simulink model "TST_TIntkVUs_VD"  (R2016b)
settings: Solver=FixedStepDiscrete  StartTime=0.0  StopTime=simTime  FixedStep=sampleTime  RelTol=1e-3
values from neighbouring files (symbols this model uses):
  testCase = 1    [initTST_TIntkVUs_VD_001.m]    (also in initTST_TIntkVUs_VD_002.m = 2; initTST_TIntkVUs_VD_003.m = 3)
libraries: UnitTest_Lib x6, simulink x4
settings Model: Creator=liangyunbo  LastModifiedBy=liangyunbo
settings DebuggingCC: SignalRangeChecking=error

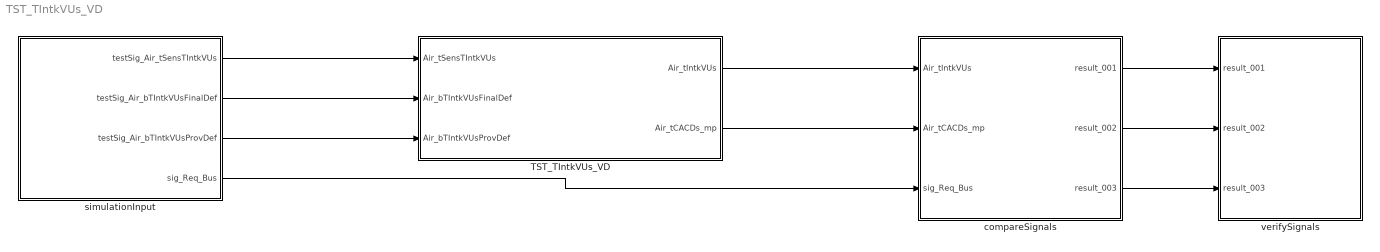
== system TST_TIntkVUs_VD ==
  TST_TIntkVUs_VD : Subsystem
  compareSignals : Subsystem
  simulationInput : Subsystem
  verifySignals : Subsystem
  wires:
  simulationInput/1(testSig_Air_tSensTIntkVUs) -> TST_TIntkVUs_VD/1(Air_tSensTIntkVUs)
  simulationInput/2(testSig_Air_bTIntkVUsFinalDef) -> TST_TIntkVUs_VD/2(Air_bTIntkVUsFinalDef)
  simulationInput/3(testSig_Air_bTIntkVUsProvDef) -> TST_TIntkVUs_VD/3(Air_bTIntkVUsProvDef)
  TST_TIntkVUs_VD/1(Air_tIntkVUs) -> compareSignals/1(Air_tIntkVUs)
  TST_TIntkVUs_VD/2(Air_tCACDs_mp) -> compareSignals/2(Air_tCACDs_mp)
  simulationInput/4(sig_Req_Bus) -> compareSignals/3(sig_Req_Bus)
  compareSignals/1(result_001) -> verifySignals/1(result_001)
  compareSignals/2(result_002) -> verifySignals/2(result_002)
  compareSignals/3(result_003) -> verifySignals/3(result_003)

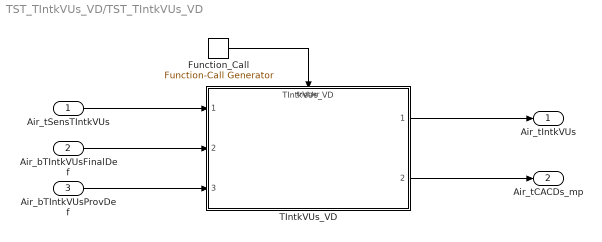
== system TST_TIntkVUs_VD/TST_TIntkVUs_VD ==
  Air_tSensTIntkVUs : Inport
  Air_bTIntkVUsFinalDef : Inport  Port=2
  Air_bTIntkVUsProvDef : Inport  Port=3
  Function_Call : simulink/Ports & Subsystems/Function-Call Generator  sample_time=sampleTime  numberOfIterations=1
  TIntkVUs_VD : ModelReference  ModelNameDialog=TIntkVUs_VD  SimulationMode=Normal  ModelReferenceVersion=1.16  TriggerPortName=function  TriggerPortTriggerType=function-call  TriggerPortStatesWhenEnabling=held
  Air_tIntkVUs : Outport
  Air_tCACDs_mp : Outport  Port=2
  wires:
  Function_Call/1 -> TIntkVUs_VD/Trigger
  Air_tSensTIntkVUs/1 -> TIntkVUs_VD/1
  Air_bTIntkVUsFinalDef/1 -> TIntkVUs_VD/2
  Air_bTIntkVUsProvDef/1 -> TIntkVUs_VD/3
  TIntkVUs_VD/1 -> Air_tIntkVUs/1
  TIntkVUs_VD/2 -> Air_tCACDs_mp/1

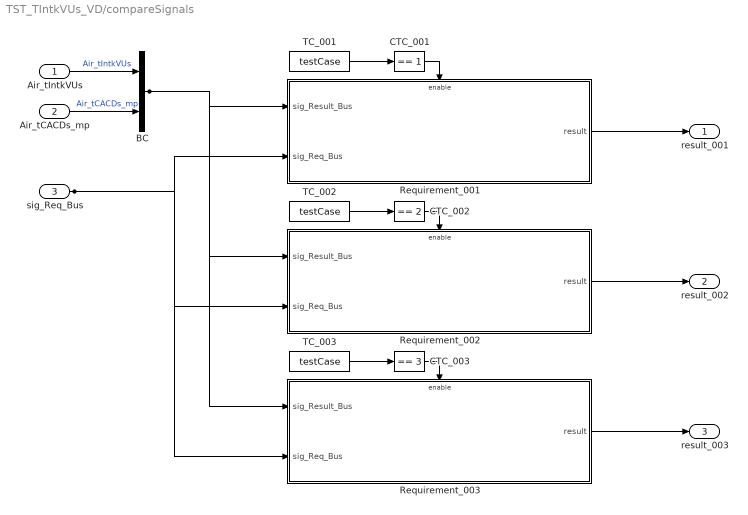
== system TST_TIntkVUs_VD/compareSignals ==
  Air_tIntkVUs : Inport
  Air_tCACDs_mp : Inport  Port=2
  sig_Req_Bus : Inport  Port=3
  BC : BusCreator  Inputs=2
  CTC_001 : simulink/Logic and Bit Operations/Compare To Constant  relop===  const=1  OutDataTypeStr=boolean
  CTC_002 : simulink/Logic and Bit Operations/Compare To Constant  relop===  const=2  OutDataTypeStr=boolean
  CTC_003 : simulink/Logic and Bit Operations/Compare To Constant  relop===  const=3  OutDataTypeStr=boolean
  Requirement_001 : Subsystem
  Requirement_002 : Subsystem
  Requirement_003 : Subsystem
  TC_001 : Constant  Value=testCase
  TC_002 : Constant  Value=testCase
  TC_003 : Constant  Value=testCase
  result_001 : Outport
  result_002 : Outport  Port=2
  result_003 : Outport  Port=3
  wires:
  Air_tIntkVUs/1 -> BC/1  "Air_tIntkVUs"
  Air_tCACDs_mp/1 -> BC/2  "Air_tCACDs_mp"
  TC_001/1 -> CTC_001/1
  CTC_001/1 -> Requirement_001/Enable
  sig_Req_Bus/1 -> Requirement_001/2(sig_Req_Bus), Requirement_002/2(sig_Req_Bus), Requirement_003/2(sig_Req_Bus)
  BC/1 -> Requirement_001/1(sig_Result_Bus), Requirement_002/1(sig_Result_Bus), Requirement_003/1(sig_Result_Bus)
  Requirement_001/1(result) -> result_001/1
  TC_002/1 -> CTC_002/1
  CTC_002/1 -> Requirement_002/Enable
  Requirement_002/1(result) -> result_002/1
  TC_003/1 -> CTC_003/1
  CTC_003/1 -> Requirement_003/Enable
  Requirement_003/1(result) -> result_003/1

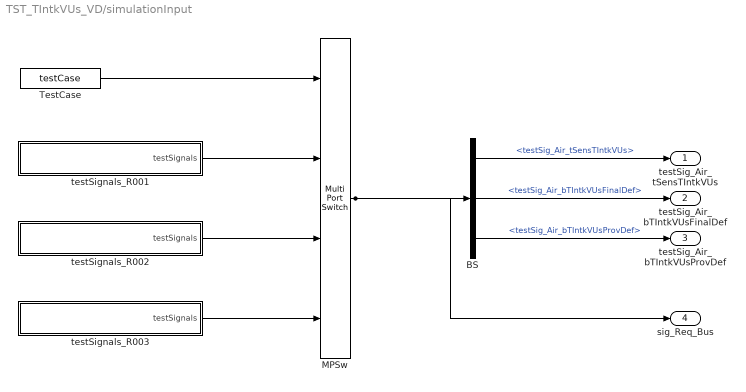
== system TST_TIntkVUs_VD/simulationInput ==
  BS : BusSelector  OutputSignals=testSig_Air_tSensTIntkVUs,testSig_Air_bTIntkVUsFinalDef,testSig_Air_bTIntkVUsProvDef
  MPSw : MultiPortSwitch  SaturateOnIntegerOverflow=on  InputSameDT=on
  TestCase : Constant  Value=testCase
  testSignals_R001 : Subsystem
  testSignals_R002 : Subsystem
  testSignals_R003 : Subsystem
  testSig_Air_tSensTIntkVUs : Outport
  testSig_Air_bTIntkVUsFinalDef : Outport  Port=2
  testSig_Air_bTIntkVUsProvDef : Outport  Port=3
  sig_Req_Bus : Outport  Port=4
  wires:
  BS/1 -> testSig_Air_tSensTIntkVUs/1  "<testSig_Air_tSensTIntkVUs>"
  BS/2 -> testSig_Air_bTIntkVUsFinalDef/1  "<testSig_Air_bTIntkVUsFinalDef>"
  BS/3 -> testSig_Air_bTIntkVUsProvDef/1  "<testSig_Air_bTIntkVUsProvDef>"
  MPSw/1 -> BS/1, sig_Req_Bus/1
  TestCase/1 -> MPSw/1
  testSignals_R001/1(testSignals) -> MPSw/2
  testSignals_R002/1(testSignals) -> MPSw/3
  testSignals_R003/1(testSignals) -> MPSw/4

== system TST_TIntkVUs_VD/verifySignals ==
  result_001 : Inport
  result_002 : Inport  Port=2
  result_003 : Inport  Port=3
  Assertion_001 : Assertion  Enabled=off
  Assertion_002 : Assertion  Enabled=off
  Assertion_003 : Assertion  Enabled=off
  wires:
  result_001/1 -> Assertion_001/1
  result_002/1 -> Assertion_002/1
  result_003/1 -> Assertion_003/1

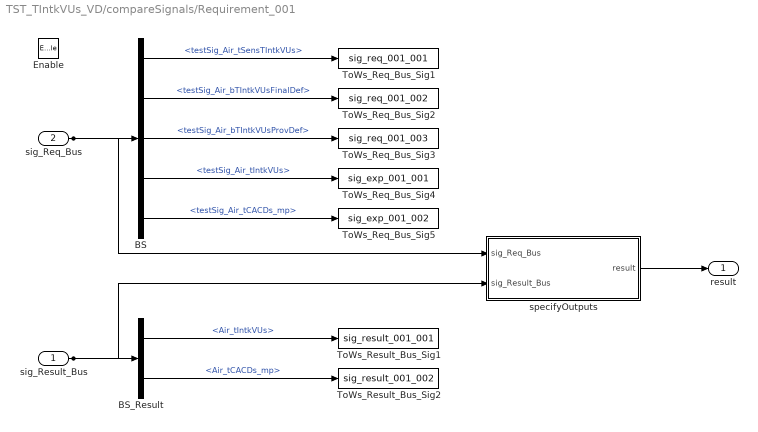
== system TST_TIntkVUs_VD/compareSignals/Requirement_001 ==
  sig_Result_Bus : Inport
  sig_Req_Bus : Inport  Port=2
  Enable : EnablePort
  BS : BusSelector  OutputSignals=testSig_Air_tSensTIntkVUs,testSig_Air_bTIntkVUsFinalDef,testSig_Air_bTIntkVUsProvDef,testSig_Air_tIntkVUs,testSig_Air_tCACDs_mp
  BS_Result : BusSelector  OutputSignals=Air_tIntkVUs,Air_tCACDs_mp
  ToWs_Req_Bus_Sig1 : ToWorkspace  VariableName=sig_req_001_001  SaveFormat=Structure With Time
  ToWs_Req_Bus_Sig2 : ToWorkspace  VariableName=sig_req_001_002  SaveFormat=Structure With Time
  ToWs_Req_Bus_Sig3 : ToWorkspace  VariableName=sig_req_001_003  SaveFormat=Structure With Time
  ToWs_Req_Bus_Sig4 : ToWorkspace  VariableName=sig_exp_001_001  SaveFormat=Structure With Time
  ToWs_Req_Bus_Sig5 : ToWorkspace  VariableName=sig_exp_001_002  SaveFormat=Structure With Time
  ToWs_Result_Bus_Sig1 : ToWorkspace  VariableName=sig_result_001_001  SaveFormat=Structure With Time
  ToWs_Result_Bus_Sig2 : ToWorkspace  VariableName=sig_result_001_002  SaveFormat=Structure With Time
  specifyOutputs : Subsystem
  result : Outport
  wires:
  sig_Req_Bus/1 -> BS/1, specifyOutputs/1(sig_Req_Bus)
  BS/1 -> ToWs_Req_Bus_Sig1/1  "<testSig_Air_tSensTIntkVUs>"
  BS/2 -> ToWs_Req_Bus_Sig2/1  "<testSig_Air_bTIntkVUsFinalDef>"
  BS/3 -> ToWs_Req_Bus_Sig3/1  "<testSig_Air_bTIntkVUsProvDef>"
  BS/4 -> ToWs_Req_Bus_Sig4/1  "<testSig_Air_tIntkVUs>"
  BS/5 -> ToWs_Req_Bus_Sig5/1  "<testSig_Air_tCACDs_mp>"
  sig_Result_Bus/1 -> BS_Result/1, specifyOutputs/2(sig_Result_Bus)
  BS_Result/1 -> ToWs_Result_Bus_Sig1/1  "<Air_tIntkVUs>"
  BS_Result/2 -> ToWs_Result_Bus_Sig2/1  "<Air_tCACDs_mp>"
  specifyOutputs/1(result) -> result/1

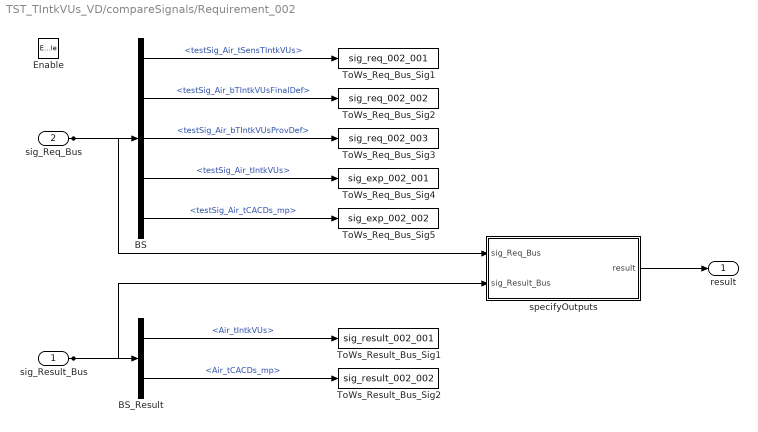
== system TST_TIntkVUs_VD/compareSignals/Requirement_002 ==
  sig_Result_Bus : Inport
  sig_Req_Bus : Inport  Port=2
  Enable : EnablePort
  BS : BusSelector  OutputSignals=testSig_Air_tSensTIntkVUs,testSig_Air_bTIntkVUsFinalDef,testSig_Air_bTIntkVUsProvDef,testSig_Air_tIntkVUs,testSig_Air_tCACDs_mp
  BS_Result : BusSelector  OutputSignals=Air_tIntkVUs,Air_tCACDs_mp
  ToWs_Req_Bus_Sig1 : ToWorkspace  VariableName=sig_req_002_001  SaveFormat=Structure With Time
  ToWs_Req_Bus_Sig2 : ToWorkspace  VariableName=sig_req_002_002  SaveFormat=Structure With Time
  ToWs_Req_Bus_Sig3 : ToWorkspace  VariableName=sig_req_002_003  SaveFormat=Structure With Time
  ToWs_Req_Bus_Sig4 : ToWorkspace  VariableName=sig_exp_002_001  SaveFormat=Structure With Time
  ToWs_Req_Bus_Sig5 : ToWorkspace  VariableName=sig_exp_002_002  SaveFormat=Structure With Time
  ToWs_Result_Bus_Sig1 : ToWorkspace  VariableName=sig_result_002_001  SaveFormat=Structure With Time
  ToWs_Result_Bus_Sig2 : ToWorkspace  VariableName=sig_result_002_002  SaveFormat=Structure With Time
  specifyOutputs : Subsystem
  result : Outport
  wires:
  sig_Req_Bus/1 -> BS/1, specifyOutputs/1(sig_Req_Bus)
  BS/1 -> ToWs_Req_Bus_Sig1/1  "<testSig_Air_tSensTIntkVUs>"
  BS/2 -> ToWs_Req_Bus_Sig2/1  "<testSig_Air_bTIntkVUsFinalDef>"
  BS/3 -> ToWs_Req_Bus_Sig3/1  "<testSig_Air_bTIntkVUsProvDef>"
  BS/4 -> ToWs_Req_Bus_Sig4/1  "<testSig_Air_tIntkVUs>"
  BS/5 -> ToWs_Req_Bus_Sig5/1  "<testSig_Air_tCACDs_mp>"
  sig_Result_Bus/1 -> BS_Result/1, specifyOutputs/2(sig_Result_Bus)
  BS_Result/1 -> ToWs_Result_Bus_Sig1/1  "<Air_tIntkVUs>"
  BS_Result/2 -> ToWs_Result_Bus_Sig2/1  "<Air_tCACDs_mp>"
  specifyOutputs/1(result) -> result/1

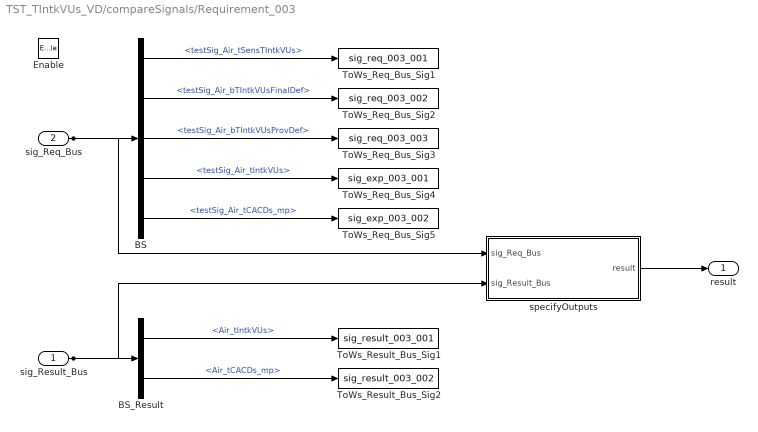
== system TST_TIntkVUs_VD/compareSignals/Requirement_003 ==
  sig_Result_Bus : Inport
  sig_Req_Bus : Inport  Port=2
  Enable : EnablePort
  BS : BusSelector  OutputSignals=testSig_Air_tSensTIntkVUs,testSig_Air_bTIntkVUsFinalDef,testSig_Air_bTIntkVUsProvDef,testSig_Air_tIntkVUs,testSig_Air_tCACDs_mp
  BS_Result : BusSelector  OutputSignals=Air_tIntkVUs,Air_tCACDs_mp
  ToWs_Req_Bus_Sig1 : ToWorkspace  VariableName=sig_req_003_001  SaveFormat=Structure With Time
  ToWs_Req_Bus_Sig2 : ToWorkspace  VariableName=sig_req_003_002  SaveFormat=Structure With Time
  ToWs_Req_Bus_Sig3 : ToWorkspace  VariableName=sig_req_003_003  SaveFormat=Structure With Time
  ToWs_Req_Bus_Sig4 : ToWorkspace  VariableName=sig_exp_003_001  SaveFormat=Structure With Time
  ToWs_Req_Bus_Sig5 : ToWorkspace  VariableName=sig_exp_003_002  SaveFormat=Structure With Time
  ToWs_Result_Bus_Sig1 : ToWorkspace  VariableName=sig_result_003_001  SaveFormat=Structure With Time
  ToWs_Result_Bus_Sig2 : ToWorkspace  VariableName=sig_result_003_002  SaveFormat=Structure With Time
  specifyOutputs : Subsystem
  result : Outport
  wires:
  sig_Req_Bus/1 -> BS/1, specifyOutputs/1(sig_Req_Bus)
  BS/1 -> ToWs_Req_Bus_Sig1/1  "<testSig_Air_tSensTIntkVUs>"
  BS/2 -> ToWs_Req_Bus_Sig2/1  "<testSig_Air_bTIntkVUsFinalDef>"
  BS/3 -> ToWs_Req_Bus_Sig3/1  "<testSig_Air_bTIntkVUsProvDef>"
  BS/4 -> ToWs_Req_Bus_Sig4/1  "<testSig_Air_tIntkVUs>"
  BS/5 -> ToWs_Req_Bus_Sig5/1  "<testSig_Air_tCACDs_mp>"
  sig_Result_Bus/1 -> BS_Result/1, specifyOutputs/2(sig_Result_Bus)
  BS_Result/1 -> ToWs_Result_Bus_Sig1/1  "<Air_tIntkVUs>"
  BS_Result/2 -> ToWs_Result_Bus_Sig2/1  "<Air_tCACDs_mp>"
  specifyOutputs/1(result) -> result/1

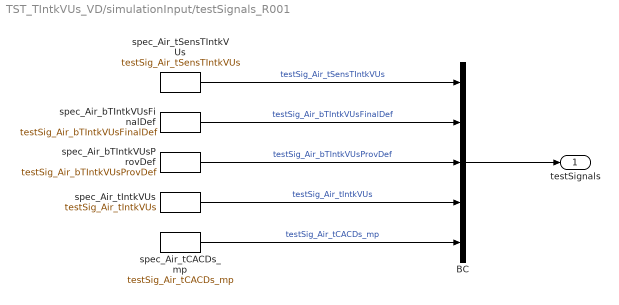
== system TST_TIntkVUs_VD/simulationInput/testSignals_R001 ==
  BC : BusCreator  Inputs=5
  spec_Air_bTIntkVUsFinalDef : FromWorkspace  VariableName=testSig_Air_bTIntkVUsFinalDef  Interpolate=off  OutputAfterFinalValue=Holding final value
  spec_Air_bTIntkVUsProvDef : FromWorkspace  VariableName=testSig_Air_bTIntkVUsProvDef  Interpolate=off  OutputAfterFinalValue=Holding final value
  spec_Air_tCACDs_mp : FromWorkspace  VariableName=testSig_Air_tCACDs_mp  Interpolate=off  OutputAfterFinalValue=Holding final value
  spec_Air_tIntkVUs : FromWorkspace  VariableName=testSig_Air_tIntkVUs  Interpolate=off  OutputAfterFinalValue=Holding final value
  spec_Air_tSensTIntkVUs : FromWorkspace  VariableName=testSig_Air_tSensTIntkVUs  Interpolate=off  OutputAfterFinalValue=Holding final value
  testSignals : Outport
  wires:
  BC/1 -> testSignals/1
  spec_Air_tSensTIntkVUs/1 -> BC/1  "testSig_Air_tSensTIntkVUs"
  spec_Air_bTIntkVUsFinalDef/1 -> BC/2  "testSig_Air_bTIntkVUsFinalDef"
  spec_Air_bTIntkVUsProvDef/1 -> BC/3  "testSig_Air_bTIntkVUsProvDef"
  spec_Air_tIntkVUs/1 -> BC/4  "testSig_Air_tIntkVUs"
  spec_Air_tCACDs_mp/1 -> BC/5  "testSig_Air_tCACDs_mp"

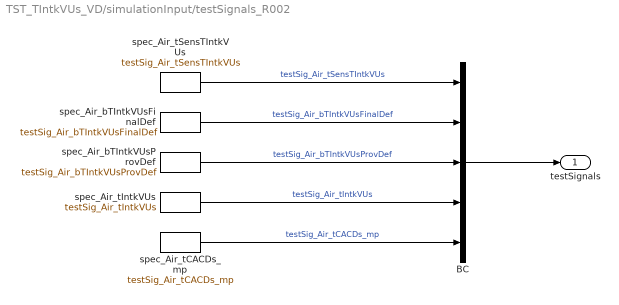
== system TST_TIntkVUs_VD/simulationInput/testSignals_R002 ==
  BC : BusCreator  Inputs=5
  spec_Air_bTIntkVUsFinalDef : FromWorkspace  VariableName=testSig_Air_bTIntkVUsFinalDef  Interpolate=off  OutputAfterFinalValue=Holding final value
  spec_Air_bTIntkVUsProvDef : FromWorkspace  VariableName=testSig_Air_bTIntkVUsProvDef  Interpolate=off  OutputAfterFinalValue=Holding final value
  spec_Air_tCACDs_mp : FromWorkspace  VariableName=testSig_Air_tCACDs_mp  Interpolate=off  OutputAfterFinalValue=Holding final value
  spec_Air_tIntkVUs : FromWorkspace  VariableName=testSig_Air_tIntkVUs  Interpolate=off  OutputAfterFinalValue=Holding final value
  spec_Air_tSensTIntkVUs : FromWorkspace  VariableName=testSig_Air_tSensTIntkVUs  Interpolate=off  OutputAfterFinalValue=Holding final value
  testSignals : Outport
  wires:
  BC/1 -> testSignals/1
  spec_Air_tSensTIntkVUs/1 -> BC/1  "testSig_Air_tSensTIntkVUs"
  spec_Air_bTIntkVUsFinalDef/1 -> BC/2  "testSig_Air_bTIntkVUsFinalDef"
  spec_Air_bTIntkVUsProvDef/1 -> BC/3  "testSig_Air_bTIntkVUsProvDef"
  spec_Air_tIntkVUs/1 -> BC/4  "testSig_Air_tIntkVUs"
  spec_Air_tCACDs_mp/1 -> BC/5  "testSig_Air_tCACDs_mp"

== system TST_TIntkVUs_VD/simulationInput/testSignals_R003 ==
  BC : BusCreator  Inputs=5
  spec_Air_bTIntkVUsFinalDef : FromWorkspace  VariableName=testSig_Air_bTIntkVUsFinalDef  Interpolate=off  OutputAfterFinalValue=Holding final value
  spec_Air_bTIntkVUsProvDef : FromWorkspace  VariableName=testSig_Air_bTIntkVUsProvDef  Interpolate=off  OutputAfterFinalValue=Holding final value
  spec_Air_tCACDs_mp : FromWorkspace  VariableName=testSig_Air_tCACDs_mp  Interpolate=off  OutputAfterFinalValue=Holding final value
  spec_Air_tIntkVUs : FromWorkspace  VariableName=testSig_Air_tIntkVUs  Interpolate=off  OutputAfterFinalValue=Holding final value
  spec_Air_tSensTIntkVUs : FromWorkspace  VariableName=testSig_Air_tSensTIntkVUs  Interpolate=off  OutputAfterFinalValue=Holding final value
  testSignals : Outport
  wires:
  BC/1 -> testSignals/1
  spec_Air_tSensTIntkVUs/1 -> BC/1  "testSig_Air_tSensTIntkVUs"
  spec_Air_bTIntkVUsFinalDef/1 -> BC/2  "testSig_Air_bTIntkVUsFinalDef"
  spec_Air_bTIntkVUsProvDef/1 -> BC/3  "testSig_Air_bTIntkVUsProvDef"
  spec_Air_tIntkVUs/1 -> BC/4  "testSig_Air_tIntkVUs"
  spec_Air_tCACDs_mp/1 -> BC/5  "testSig_Air_tCACDs_mp"

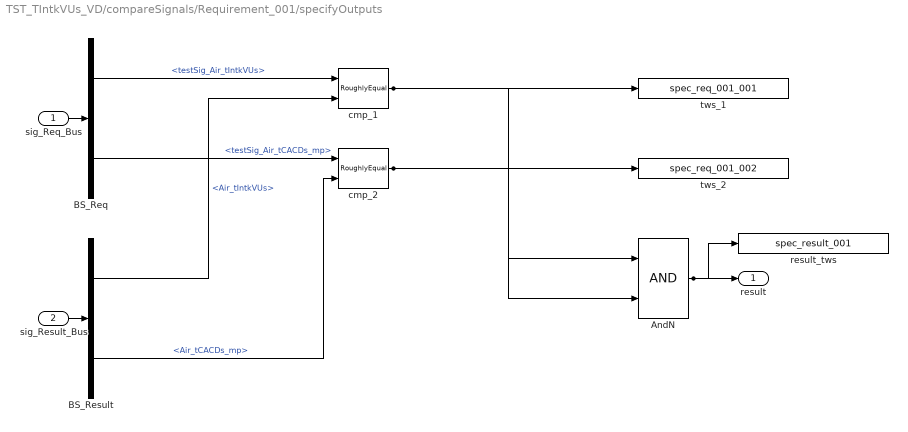
== system TST_TIntkVUs_VD/compareSignals/Requirement_001/specifyOutputs ==
  sig_Req_Bus : Inport
  sig_Result_Bus : Inport  Port=2
  AndN : Logic
  BS_Req : BusSelector  OutputSignals=testSig_Air_tIntkVUs,testSig_Air_tCACDs_mp
  BS_Result : BusSelector  OutputSignals=Air_tIntkVUs,Air_tCACDs_mp
  cmp_1 : UnitTest_Lib/RoughlyEqual  slope=0.1
  cmp_2 : UnitTest_Lib/RoughlyEqual  slope=0.1
  result_tws : ToWorkspace  VariableName=spec_result_001
  tws_1 : ToWorkspace  VariableName=spec_req_001_001
  tws_2 : ToWorkspace  VariableName=spec_req_001_002
  result : Outport
  wires:
  sig_Req_Bus/1 -> BS_Req/1
  sig_Result_Bus/1 -> BS_Result/1
  AndN/1 -> result/1, result_tws/1
  BS_Req/1 -> cmp_1/1  "<testSig_Air_tIntkVUs>"
  BS_Result/1 -> cmp_1/2  "<Air_tIntkVUs>"
  cmp_1/1 -> tws_1/1, AndN/1
  BS_Req/2 -> cmp_2/1  "<testSig_Air_tCACDs_mp>"
  BS_Result/2 -> cmp_2/2  "<Air_tCACDs_mp>"
  cmp_2/1 -> tws_2/1, AndN/2

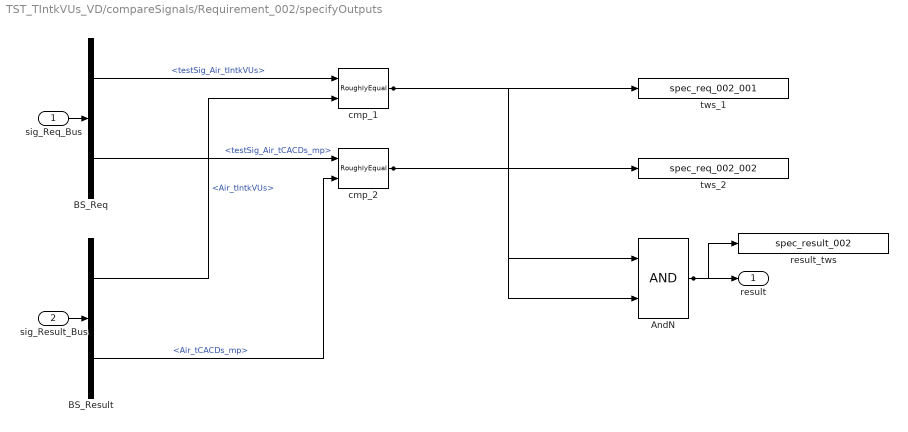
== system TST_TIntkVUs_VD/compareSignals/Requirement_002/specifyOutputs ==
  sig_Req_Bus : Inport
  sig_Result_Bus : Inport  Port=2
  AndN : Logic
  BS_Req : BusSelector  OutputSignals=testSig_Air_tIntkVUs,testSig_Air_tCACDs_mp
  BS_Result : BusSelector  OutputSignals=Air_tIntkVUs,Air_tCACDs_mp
  cmp_1 : UnitTest_Lib/RoughlyEqual  slope=0.1
  cmp_2 : UnitTest_Lib/RoughlyEqual  slope=0.1
  result_tws : ToWorkspace  VariableName=spec_result_002
  tws_1 : ToWorkspace  VariableName=spec_req_002_001
  tws_2 : ToWorkspace  VariableName=spec_req_002_002
  result : Outport
  wires:
  sig_Req_Bus/1 -> BS_Req/1
  sig_Result_Bus/1 -> BS_Result/1
  AndN/1 -> result/1, result_tws/1
  BS_Req/1 -> cmp_1/1  "<testSig_Air_tIntkVUs>"
  BS_Result/1 -> cmp_1/2  "<Air_tIntkVUs>"
  cmp_1/1 -> tws_1/1, AndN/1
  BS_Req/2 -> cmp_2/1  "<testSig_Air_tCACDs_mp>"
  BS_Result/2 -> cmp_2/2  "<Air_tCACDs_mp>"
  cmp_2/1 -> tws_2/1, AndN/2

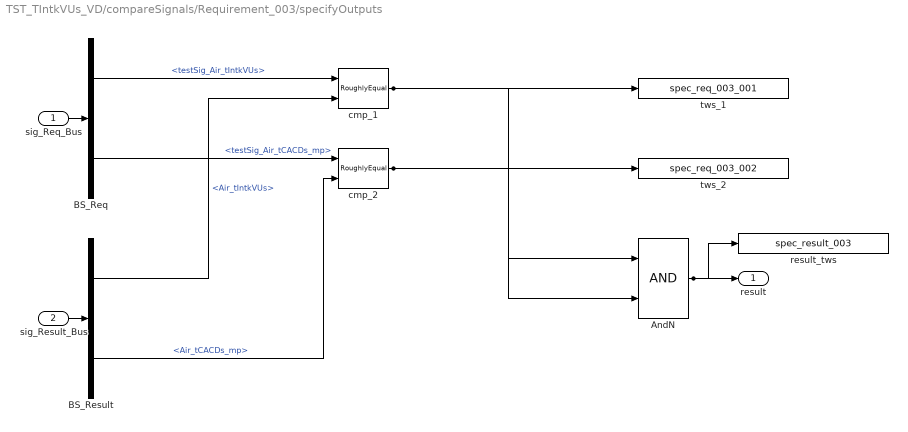
== system TST_TIntkVUs_VD/compareSignals/Requirement_003/specifyOutputs ==
  sig_Req_Bus : Inport
  sig_Result_Bus : Inport  Port=2
  AndN : Logic
  BS_Req : BusSelector  OutputSignals=testSig_Air_tIntkVUs,testSig_Air_tCACDs_mp
  BS_Result : BusSelector  OutputSignals=Air_tIntkVUs,Air_tCACDs_mp
  cmp_1 : UnitTest_Lib/RoughlyEqual  slope=0.1
  cmp_2 : UnitTest_Lib/RoughlyEqual  slope=0.1
  result_tws : ToWorkspace  VariableName=spec_result_003
  tws_1 : ToWorkspace  VariableName=spec_req_003_001
  tws_2 : ToWorkspace  VariableName=spec_req_003_002
  result : Outport
  wires:
  sig_Req_Bus/1 -> BS_Req/1
  sig_Result_Bus/1 -> BS_Result/1
  AndN/1 -> result/1, result_tws/1
  BS_Req/1 -> cmp_1/1  "<testSig_Air_tIntkVUs>"
  BS_Result/1 -> cmp_1/2  "<Air_tIntkVUs>"
  cmp_1/1 -> tws_1/1, AndN/1
  BS_Req/2 -> cmp_2/1  "<testSig_Air_tCACDs_mp>"
  BS_Result/2 -> cmp_2/2  "<Air_tCACDs_mp>"
  cmp_2/1 -> tws_2/1, AndN/2
